simulink model "busilica"  (R2024a)
settings: Solver=VariableStepAuto  StartTime=0.0  StopTime=Tspan  RelTol=1e-3
values from neighbouring files (symbols this model uses):
  c = 400    [glavni_kod.m]    (also in pocetnigraf.m)
  d = 20    [glavni_kod.m]    (also in pocetnigraf.m)
  ip = 12.5    [glavni_kod.m]    (also in pocetnigraf.m)
  J1 = 10    [glavni_kod.m]    (also in pocetnigraf.m)
  J2 = 640    [glavni_kod.m]    (also in pocetnigraf.m)
  Td = 0.5    [glavni_kod.m]    (also in pocetnigraf.m)
undefined symbols (not defined in the file or in its folder): kontroler
settings Model: Creator=Martin  LastModifiedBy=Marko
settings DataIOCC: ReturnWorkspaceOutputs=off

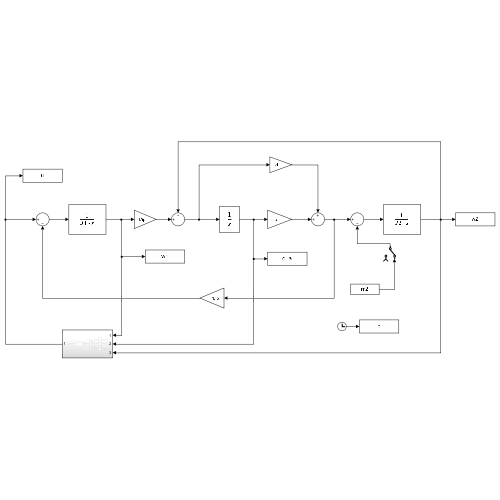
[thumbnail: Simulink's stored preview of the top-level diagram]
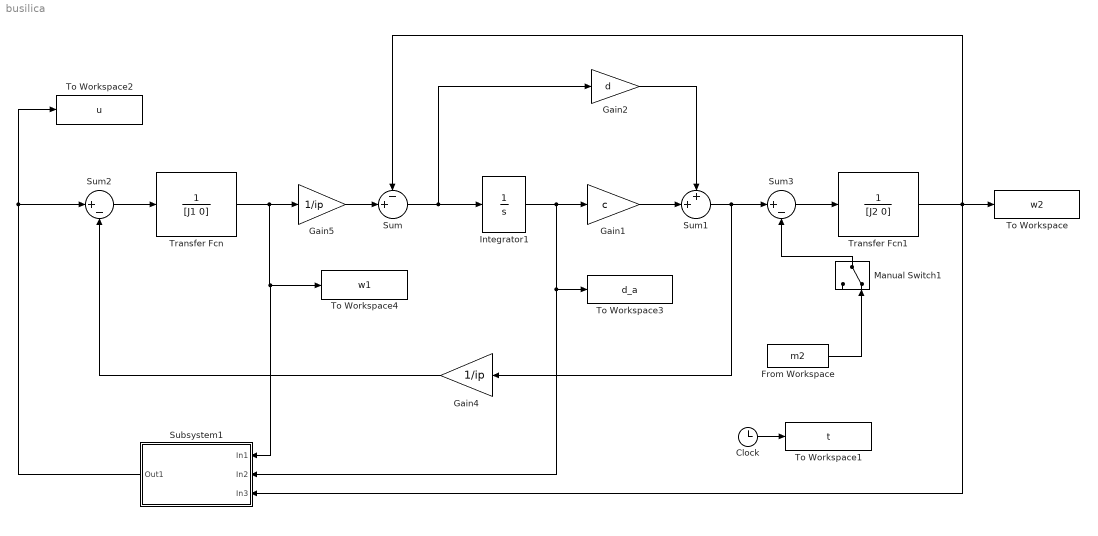
== system busilica ==
  Clock : Clock
  From Workspace : FromWorkspace  VariableName=m2
  Gain1 : Gain  Gain=c
  Gain2 : Gain  Gain=d
  Gain4 : Gain  Gain=1/ip
  Gain5 : Gain  Gain=1/ip
  Integrator1 : Integrator
  Manual Switch1 : ManualSwitch  CurrentSetting=0
  Subsystem1 : Subsystem
  Sum : Sum  Inputs=-+|
  Sum1 : Sum  Inputs=++|
  Sum2 : Sum  Inputs=|+-
  Sum3 : Sum  Inputs=|+-
  To Workspace : ToWorkspace  VariableName=w2  SampleTime=Td
  To Workspace1 : ToWorkspace  VariableName=t  SampleTime=Td
  To Workspace2 : ToWorkspace  VariableName=u  SampleTime=Td
  To Workspace3 : ToWorkspace  VariableName=d_a  SampleTime=Td
  To Workspace4 : ToWorkspace  VariableName=w1  SampleTime=Td
  Transfer Fcn : TransferFcn  Denominator=[J1 0]
  Transfer Fcn1 : TransferFcn  Denominator=[J2 0]
  wires:
  From Workspace/1 -> Manual Switch1/2
  Integrator1/1 -> Gain1/1, To Workspace3/1, Subsystem1/2(In2)
  Gain2/1 -> Sum1/1
  Sum/1 -> Integrator1/1, Gain2/1
  Transfer Fcn1/1 -> To Workspace/1, Sum/1, Subsystem1/3(In3)
  Transfer Fcn/1 -> Subsystem1/1(In1), To Workspace4/1, Gain5/1
  Clock/1 -> To Workspace1/1
  Gain4/1 -> Sum2/2
  Sum1/1 -> Sum3/1, Gain4/1
  Manual Switch1/1 -> Sum3/2
  Sum3/1 -> Transfer Fcn1/1
  Subsystem1/1(Out1) -> To Workspace2/1, Sum2/1
  Sum2/1 -> Transfer Fcn/1
  Gain5/1 -> Sum/2
  Gain1/1 -> Sum1/2

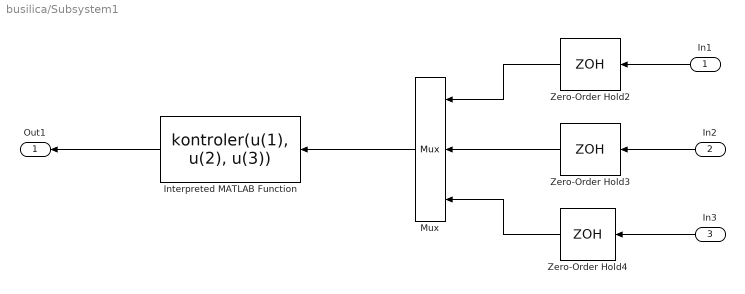
== system busilica/Subsystem1 ==
  In1 : Inport
  In2 : Inport  Port=2
  In3 : Inport  Port=3
  Interpreted MATLAB Function : MATLABFcn  MATLABFcn=kontroler(u(1), u(2), u(3))  OutputDimensions=m
  Mux : Mux  Inputs=3
  Zero-Order Hold2 : ZeroOrderHold  SampleTime=Td
  Zero-Order Hold3 : ZeroOrderHold  SampleTime=Td
  Zero-Order Hold4 : ZeroOrderHold  SampleTime=Td
  Out1 : Outport
  wires:
  Interpreted MATLAB Function/1 -> Out1/1
  Zero-Order Hold2/1 -> Mux/1
  Mux/1 -> Interpreted MATLAB Function/1
  Zero-Order Hold3/1 -> Mux/2
  Zero-Order Hold4/1 -> Mux/3
  In1/1 -> Zero-Order Hold2/1
  In2/1 -> Zero-Order Hold3/1
  In3/1 -> Zero-Order Hold4/1
